simulink model "c2000_host_read_12M"  (R2021b)
settings: Solver=FixedStepDiscrete  StartTime=0.0  StopTime=inf  RelTol=1e-3  EnableMultiTasking=on
libraries: instrumentseriallib x3, demo_controls x1
settings Model: Creator=The MathWorks, Inc.  LastModifiedBy=The MathWorks, Inc.
settings SolverCC: AlgebraicLoopSolver=TrustRegion
settings DataIOCC: LimitDataPoints=on  SaveFormat=Array  ReturnWorkspaceOutputs=off
settings OptimizationCC: LifeSpan=1  EfficientTunableParamExpr=on
settings DebuggingCC: UnderspecifiedInitializationDetection=Classic  MergeDetectMultiDrivingBlocksExec=none  SolverPrmCheckMsg=warning  AllowSymbolicDim=off  SFUnexpectedBacktrackingDiag=warning  SFNoUnconditionalDefaultTransitionDiag=warning  SFExecutionAtInitializationDiag=none  SFMachineParentedDataDiag=warning  ArithmeticOperatorsInVariantConditions=warning
settings HardwareCC: ProdBitPerPointer=32  ProdBitPerSizeT=32  ProdBitPerPtrDiffT=32  ProdLargestAtomicFloat=None  ProdIntDivRoundTo=Undefined  ProdEndianess=Unspecified  ProdWordSize=32  ProdHWDeviceType=32-bit Generic
settings ModelReferenceCC: PropagateSignalLabelsOutOfModel=off
settings SFSimCC: SimUseLocalCustomCode=off  MATLABDynamicMemAlloc=off  CustomCodeUndefinedFunction=UseInterfaceOnly
settings RTWCC: Description=Real-Time Workshop Embedded Coder  SystemTargetFile=ert.tlc  TemplateMakefile=ert_default_tmf  GenerateReport=on  RTWUseLocalCustomCode=off  IncludeHyperlinkInReport=on  LaunchReport=on  GenerateTraceInfo=on  GenerateTraceReport=on  GenerateTraceReportSl=on  GenerateTraceReportSf=on  GenerateTraceReportEml=on
settings CodeAppCC: IgnoreCustomStorageClasses=off  CustomSymbolStrModelFcn=$N  StateflowObjectComments=on  InternalIdentifier=Classic
settings ERTTargetCC: MultiwordLength=2048  GenerateSampleERTMain=on  ERTCustomFileTemplate=example_file_process.tlc  ConvertIfToSwitch=off  SuppressUnreachableDefaultCases=off
settings ConfigComp: CovMetricSettings=dw  CovSaveCumulativeToWorkspaceVar=on  CovSaveSingleToWorkspaceVar=on  CovExternalEMLEnable=off  CovSFcnEnable=off

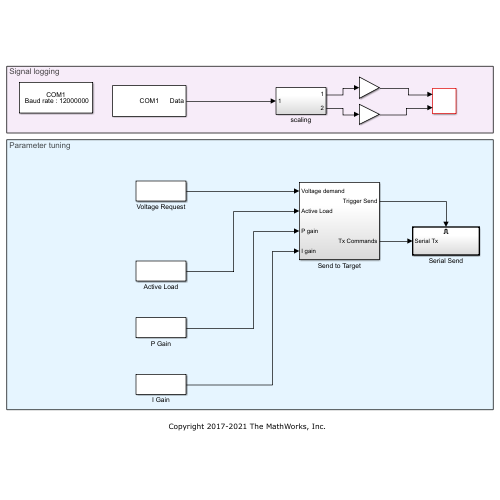
[thumbnail: Simulink's stored preview of the top-level diagram]
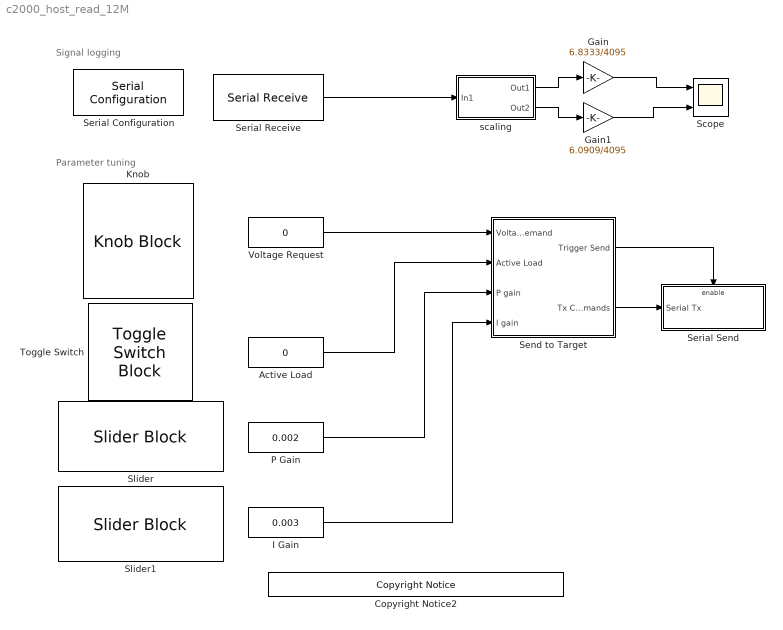
== system c2000_host_read_12M ==
  note: Parameter tuning
  note: Signal logging
  Active Load : Constant  Value=0  VectorParams1D=off  OutDataTypeStr=uint16  SampleTime=.06
  Copyright Notice2 : demo_controls/Copyright Notice  year=2017  prod=tic2000
      settings: SourceProductBaseCode=ME
  Gain : Gain  Gain=6.8333/4095
  Gain1 : Gain  Gain=6.0909/4095
  I Gain : Constant  Value=0.003  VectorParams1D=off  OutDataTypeStr=single  SampleTime=.06
  Knob : KnobBlock  ScaleMax=6
  P Gain : Constant  Value=0.002  VectorParams1D=off  OutDataTypeStr=single  SampleTime=.06
  Scope : Scope  NumInputPorts=2
  Send to Target : Subsystem
  Serial Configuration : instrumentseriallib/Serial Configuration  Priority=-200000  Port=COM1  ComPort=<Select a port...>  BaudRate=12000000  DataBits=8  Parity=none  StopBits=1  ByteOrder=little-endian  FlowControl=hardware  Timeout=2  SimulateUsing=Interpreted execution  BlockInModel=on
  Serial Receive : instrumentseriallib/Serial Receive  Port=COM1  ComPort=COM1  DataType=uint16  SaveDataType=uint8  ToggleHeader=on  Header="[ 83  83 ]"  ToggleTerminator=on  Terminator=Custom terminator  CustomTerminator="[ 69  69 ]"  ToggleDataSize=on  DataSize="[2  12000]"  EnableBlockingMode=on  ActionDataUnavailable=Output last received value  ActionWhenDataUnavailable=Output last received value  CustomValue=0  SampleTime=0.06  SimulateUsing=Interpreted execution  BlockInModel=on
  Serial Send : Subsystem  TreatAsAtomicUnit=on
  Slider : SliderBlock  ScaleMax=0.10000000000000001
  Slider1 : SliderBlock  ScaleMax=0.10000000000000001
  Toggle Switch : ToggleSwitchBlock
      settings: Values={{'Off', 'On'}, [0 1]}
  Voltage Request : Constant  Value=0  VectorParams1D=off  OutDataTypeStr=single  SampleTime=0.06
  scaling : Subsystem
  wires:
  Voltage Request/1 -> Send to Target/1(Voltage demand)
  Active Load/1 -> Send to Target/2(Active Load)
  P Gain/1 -> Send to Target/3(P gain)
  I Gain/1 -> Send to Target/4(I gain)
  Serial Receive/1 -> scaling/1(In1)
  scaling/1(Out1) -> Gain/1
  Send to Target/1(Trigger Send) -> Serial Send/Enable
  Send to Target/2(Tx Commands) -> Serial Send/1(Serial Tx)
  Gain/1 -> Scope/1
  scaling/2(Out2) -> Gain1/1
  Gain1/1 -> Scope/2

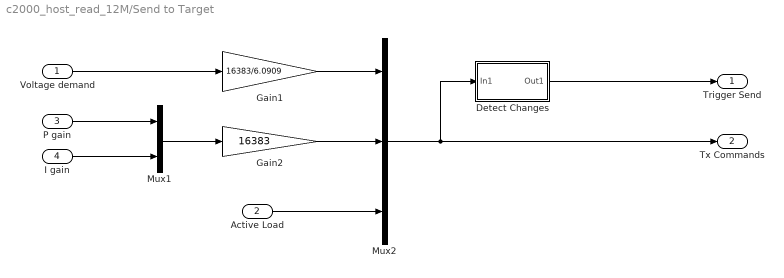
== system c2000_host_read_12M/Send to Target ==
  Voltage demand : Inport
  Active Load : Inport  Port=2
  P gain : Inport  Port=3
  I gain : Inport  Port=4
  Detect Changes : Subsystem
  Gain1 : Gain  Gain=16383/6.0909  OutDataTypeStr=uint16
  Gain2 : Gain  Gain=16383  OutDataTypeStr=uint16
  Mux1 : Mux  Inputs=2
  Mux2 : Mux  Inputs=3
  Trigger Send : Outport  VectorParamsAs1DForOutWhenUnconnected=off
  Tx Commands : Outport  Port=2  VectorParamsAs1DForOutWhenUnconnected=off
  wires:
  Voltage demand/1 -> Gain1/1
  Active Load/1 -> Mux2/3
  P gain/1 -> Mux1/1
  Mux1/1 -> Gain2/1
  Gain2/1 -> Mux2/2
  Mux2/1 -> Detect Changes/1(In1), Tx Commands/1
  Detect Changes/1(Out1) -> Trigger Send/1
  I gain/1 -> Mux1/2
  Gain1/1 -> Mux2/1

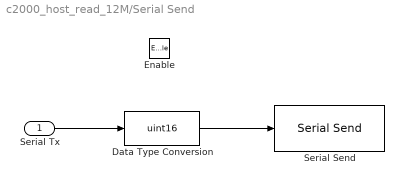
== system c2000_host_read_12M/Serial Send ==
  Serial Tx : Inport
  Enable : EnablePort
  Data Type Conversion : DataTypeConversion  OutDataTypeStr=uint16  ConvertRealWorld=Stored Integer (SI)
  Serial Send : instrumentseriallib/Serial Send  Port=COM1  ComPort=COM1  Header=[ 83 ]  Terminator=Custom terminator  CustomTerminator=[ 69 ]  EnableBlockingMode=off  SimulateUsing=Interpreted execution  BlockInModel=on
  wires:
  Data Type Conversion/1 -> Serial Send/1
  Serial Tx/1 -> Data Type Conversion/1

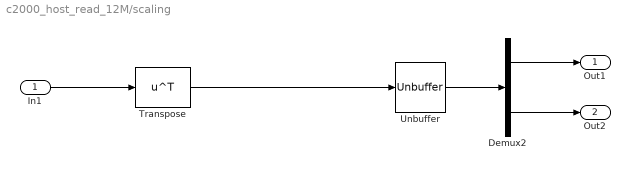
== system c2000_host_read_12M/scaling ==
  In1 : Inport
  Demux2 : Demux  Outputs=2
  Transpose : Math  Operator=transpose  SignedPower=on  SaturateOnIntegerOverflow=on
  Unbuffer : Unbuffer
  Out1 : Outport  VectorParamsAs1DForOutWhenUnconnected=off
  Out2 : Outport  Port=2  VectorParamsAs1DForOutWhenUnconnected=off
  wires:
  In1/1 -> Transpose/1
  Unbuffer/1 -> Demux2/1
  Demux2/1 -> Out1/1
  Demux2/2 -> Out2/1
  Transpose/1 -> Unbuffer/1

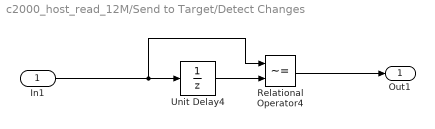
== system c2000_host_read_12M/Send to Target/Detect Changes ==
  In1 : Inport
  Relational Operator4 : RelationalOperator  Operator=~=  OutDataTypeStr=boolean  RndMeth=Nearest
  Unit Delay4 : UnitDelay  SampleTime=-1  HasFrameUpgradeWarning=on
  Out1 : Outport  VectorParamsAs1DForOutWhenUnconnected=off
  wires:
  Unit Delay4/1 -> Relational Operator4/2
  In1/1 -> Relational Operator4/1, Unit Delay4/1
  Relational Operator4/1 -> Out1/1
